simulink model "six_plus_six_AcmsteeringV09_main_2lfrf"  (R2014a)
settings: Solver=FixedStepDiscrete  StartTime=0.0  StopTime=10.0  FixedStep=0.0005  RelTol=1e-3
InitFcn:
  | Veh_Par_wxt
undefined symbols (not defined in the file or in its folder): acc_spdctl, ag_thr, B, bra_em, bra_pre_gz2, bra_pre_gz34, bra_pre_yd, brakepre_dem_data, brakeTrq_dem_data, bratrq_max, ecucoder_acal, eff_tran, ESP_switch, G, guzhang_lf, guzhang_lm, guzhang_lr, guzhang_rf, guzhang_rm, guzhang_rr, kd1, kd2, ki1, ki2, kp1, kp2, L, myFIS, premax, Radius, RC_switch, s_opt_yi, s_opt_zhuan, s_opt_zhuan_add, s_opt_zhuan_table, spd_map_mot, spd_spdctl, speed_thr_park, TCS_switch, tras_ratio, trq_map_mot, trqmax_yd, trqmax_zx, trqmaxneg, v_gain, v_table, v_thr_park, zhidong_bianmazhi, zhidong_down, zhidong_up, zhidong_youmen, zhuanxiang_bianmazhi, zhuanxiang_down, zhuanxiang_up, zhuanxiang_youmen
libraries: simulink x980, ec5744lib x59, fuzblock x2
(part 25 of 25)

== matlab function six_plus_six_AcmsteeringV09_main_2lfrf/MainControl/mode_control/forward/forward/Drive/容错控制/MATLAB Function ==
  data: trq_dem_l input; trq_dem_lf output; trq_dem_lm output; trq_dem_r input; trqlim_lf input; trqlim_lm input; trqlim_lr input; trqlim_rf input; trqlim_rm input; trqlim_rr input; guzhang_lf input; guzhang_lm input; guzhang_lr input; guzhang_rf input; guzhang_rm input; guzhang_rr input; trq_dem_lr output; trq_dem_rf output; trq_dem_rm output; trq_dem_rr output; bra_pre_l output; bra_pre_r output; bra_pre_gz2 input; bra_pre_gz34 input; mode output int8
function [trq_dem_lf,trq_dem_lm,trq_dem_lr,trq_dem_rf,trq_dem_rm,trq_dem_rr,bra_pre_l,bra_pre_r,mode] = fcn(trq_dem_l,trq_dem_r,trqlim_lf,trqlim_lm,trqlim_lr,trqlim_rf,trqlim_rm,trqlim_rr,guzhang_lf,guzhang_lm,guzhang_lr,guzhang_rf,guzhang_rm,guzhang_rr,bra_pre_gz2,bra_pre_gz34)
%#codegen
if guzhang_lf==0 && guzhang_lm==0 && guzhang_lr==0 && guzhang_rf==0 && guzhang_rm==0 && guzhang_rr==0    %0电机故障,平均分配
    trq_dem_lf=single(trq_dem_l/3);
    trq_dem_lm=single(trq_dem_l/3);
    trq_dem_lr=single(trq_dem_l/3);
    trq_dem_rf=single(trq_dem_r/3);
    trq_dem_rm=single(trq_dem_r/3);
    trq_dem_rr=single(trq_dem_r/3);
    bra_pre_l=single(0);
    bra_pre_r=single(0);
    mode=int8(1);
    
    
    
    
elseif guzhang_lf==1 && guzhang_lm==0 && guzhang_lr==0 && guzhang_rf==0 && guzhang_rm==0 && guzhang_rr==0    %1电机故障，同侧电机进行力矩转移，超过限值后，对侧亦降扭。  左前
    trq_dem_lf=single(0);
    trq_dem_lm=single(min(trq_dem_l/2,trqlim_lm));
    trq_dem_lr=single(min(trq_dem_l/2,trqlim_lr));
    trq_dem_rf=single((trq_dem_r-(trq_dem_l-trq_dem_lm-trq_dem_lr))/3);
    trq_dem_rm=single((trq_dem_r-(trq_dem_l-trq_dem_lm-trq_dem_lr))/3);
    trq_dem_rr=single((trq_dem_r-(trq_dem_l-trq_dem_lm-trq_dem_lr))/3);
    bra_pre_l=single(0);
    bra_pre_r=single(0);
    mode=int8(2);
elseif guzhang_lf==0 && guzhang_lm==1 && guzhang_lr==0 && guzhang_rf==0 && guzhang_rm==0 && guzhang_rr==0    %1电机故障，同侧电机进行力矩转移，超过限值后，对侧亦降扭。 左中
    trq_dem_lf=single(min(trq_dem_l/2,trqlim_lf));
    trq_dem_lm=single(0);
    trq_dem_lr=single(min(trq_dem_l/2,trqlim_lr));
    trq_dem_rf=single((trq_dem_r-(trq_dem_l-trq_dem_lf-trq_dem_lr))/3);
    trq_dem_rm=single((trq_dem_r-(trq_dem_l-trq_dem_lf-trq_dem_lr))/3);
    trq_dem_rr=single((trq_dem_r-(trq_dem_l-trq_dem_lf-trq_dem_lr))/3);
    bra_pre_l=single(0);
    bra_pre_r=single(0);
    mode=int8(3);
elseif guzhang_lf==0 && guzhang_lm==0 && guzhang_lr==1 && guzhang_rf==0 && guzhang_rm==0 && guzhang_rr==0    %1电机故障，同侧电机进行力矩转移，超过限值后，对侧亦降扭。 左后
    trq_dem_lf=single(min(trq_dem_l/2,trqlim_lf));
    trq_dem_lm=single(min(trq_dem_l/2,trqlim_lm));
    trq_dem_lr=single(0);
    trq_dem_rf=single((trq_dem_r-(trq_dem_l-trq_dem_lf-trq_dem_lm))/3);
    trq_dem_rm=single((trq_dem_r-(trq_dem_l-trq_dem_lf-trq_dem_lm))/3);
    trq_dem_rr=single((trq_dem_r-(trq_dem_l-trq_dem_lf-trq_dem_lm))/3);
    bra_pre_l=single(0);
    bra_pre_r=single(0);
    mode=int8(4);
elseif guzhang_lf==0 && guzhang_lm==0 && guzhang_lr==0 && guzhang_rf==1 && guzhang_rm==0 && guzhang_rr==0    %1电机故障，同侧电机进行力矩转移，超过限值后，对侧亦降扭。  右前
    trq_dem_rf=single(0);
    trq_dem_rm=single(min(trq_dem_r/2,trqlim_rm));
    trq_dem_rr=single(min(trq_dem_r/2,trqlim_rr));
    trq_dem_lf=single((trq_dem_l-(trq_dem_r-trq_dem_rm-trq_dem_rr))/3);
    trq_dem_lm=single((trq_dem_l-(trq_dem_r-trq_dem_rm-trq_dem_rr))/3);
    trq_dem_lr=single((trq_dem_l-(trq_dem_r-trq_dem_rm-trq_dem_rr))/3);
    bra_pre_l=single(0);
    bra_pre_r=single(0);
    mode=int8(5);
elseif guzhang_lf==0 && guzhang_lm==0 && guzhang_lr==0 && guzhang_rf==0 && guzhang_rm==1 && guzhang_rr==0    %1电机故障，同侧电机进行力矩转移，超过限值后，对侧亦降扭。 右中
    trq_dem_rf=single(min(trq_dem_r/2,trqlim_rf));
    trq_dem_rm=single(0);
    trq_dem_rr=single(min(trq_dem_r/2,trqlim_rr));
    trq_dem_lf=single((trq_dem_l-(trq_dem_r-trq_dem_rf-trq_dem_rr))/3);
    trq_dem_lm=single((trq_dem_l-(trq_dem_r-trq_dem_rf-trq_dem_rr))/3);
    trq_dem_lr=single((trq_dem_l-(trq_dem_r-trq_dem_rf-trq_dem_rr))/3);
    bra_pre_l=single(0);
    bra_pre_r=single(0);
    mode=int8(6);
elseif guzhang_lf==0 && guzhang_lm==0 && guzhang_lr==0 && guzhang_rf==0 && guzhang_rm==0 && guzhang_rr==1    %1电机故障，同侧电机进行力矩转移，超过限值后，对侧亦降扭。 右后
    trq_dem_rf=single(min(trq_dem_r/2,trqlim_rf));
    trq_dem_rm=single(min(trq_dem_r/2,trqlim_rm));
    trq_dem_rr=single(0);
    trq_dem_lf=single((trq_dem_l-(trq_dem_r-trq_dem_rf-trq_dem_rm))/3);
    trq_dem_lm=single((trq_dem_l-(trq_dem_r-trq_dem_rf-trq_dem_rm))/3);
    trq_dem_lr=single((trq_dem_l-(trq_dem_r-trq_dem_rf-trq_dem_rm))/3);
    bra_pre_l=single(0);
    bra_pre_r=single(0);
    mode=int8(7);
    
    
    
    
    
    
elseif guzhang_lf==1 && guzhang_lm==1 && guzhang_lr==0 && guzhang_rf==0 && guzhang_rm==0 && guzhang_rr==0    %2电机故障，同侧电机进行力矩转移，超过限值后，对侧亦降扭。  左前 左中   左侧
    trq_dem_lf=single(0);
    trq_dem_lm=single(0);
    trq_dem_lr=single(min(trq_dem_l,trqlim_lr));
    trq_dem_rf=single((trq_dem_r-(trq_dem_l-trq_dem_lr))/3);
    trq_dem_rm=single((trq_dem_r-(trq_dem_l-trq_dem_lr))/3);
    trq_dem_rr=single((trq_dem_r-(trq_dem_l-trq_dem_lr))/3);
    bra_pre_l=single(0);
    bra_pre_r=single(0);
    mode=int8(8);
elseif guzhang_lf==1 && guzhang_lm==0 && guzhang_lr==1 && guzhang_rf==0 && guzhang_rm==0 && guzhang_rr==0    %2电机故障，同侧电机进行力矩转移，超过限值后，对侧亦降扭。  左前 左后
    trq_dem_lf=single(0);
    trq_dem_lm=single(min(trq_dem_l,trqlim_lm));
    trq_dem_lr=single(0);
    trq_dem_rf=single((trq_dem_r-(trq_dem_l-trq_dem_lm))/3);
    trq_dem_rm=single((trq_dem_r-(trq_dem_l-trq_dem_lm))/3);
    trq_dem_rr=single((trq_dem_r-(trq_dem_l-trq_dem_lm))/3);
    bra_pre_l=single(0);
    bra_pre_r=single(0);
    mode=int8(9);
elseif guzhang_lf==0 && guzhang_lm==1 && guzhang_lr==1 && guzhang_rf==0 && guzhang_rm==0 && guzhang_rr==0    %2电机故障，同侧电机进行力矩转移，超过限值后，对侧亦降扭。  左中 左后
    trq_dem_lf=single(min(trq_dem_l,trqlim_lf));
    trq_dem_lm=single(0);
    trq_dem_lr=single(0);
    trq_dem_rf=single((trq_dem_r-(trq_dem_l-trq_dem_lf))/3);
    trq_dem_rm=single((trq_dem_r-(trq_dem_l-trq_dem_lf))/3);
    trq_dem_rr=single((trq_dem_r-(trq_dem_l-trq_dem_lf))/3);
    bra_pre_l=single(0);
    bra_pre_r=single(0);
    mode=int8(10);
    
elseif guzhang_lf==0 && guzhang_lm==0 && guzhang_lr==0 && guzhang_rf==1 && guzhang_rm==1 && guzhang_rr==0    %2电机故障，同侧电机进行力矩转移，超过限值后，对侧亦降扭。  右前 右中   右侧
    trq_dem_rf=single(0);
    trq_dem_rm=single(0);
    trq_dem_rr=single(min(trq_dem_r,trqlim_rr));
    trq_dem_lf=single((trq_dem_l-(trq_dem_r-trq_dem_rr))/3);
    trq_dem_lm=single((trq_dem_l-(trq_dem_r-trq_dem_rr))/3);
    trq_dem_lr=single((trq_dem_l-(trq_dem_r-trq_dem_rr))/3);
    bra_pre_l=single(0);
    bra_pre_r=single(0);
    mode=int8(11);
elseif guzhang_lf==0 && guzhang_lm==0 && guzhang_lr==0 && guzhang_rf==1 && guzhang_rm==0 && guzhang_rr==1    %2电机故障，同侧电机进行力矩转移，超过限值后，对侧亦降扭。  右前 右后
    trq_dem_rf=single(0);
    trq_dem_rm=single(min(trq_dem_r,trqlim_rm));
    trq_dem_rr=single(0);
    trq_dem_lf=single((trq_dem_l-(trq_dem_r-trq_dem_rm))/3);
    trq_dem_lm=single((trq_dem_l-(trq_dem_r-trq_dem_rm))/3);
    trq_dem_lr=single((trq_dem_l-(trq_dem_r-trq_dem_rm))/3);
    bra_pre_l=single(0);
    bra_pre_r=single(0);
    mode=int8(12);
elseif guzhang_lf==0 && guzhang_lm==0 && guzhang_lr==0 && guzhang_rf==0 && guzhang_rm==1 && guzhang_rr==1    %2电机故障，同侧电机进行力矩转移，超过限值后，对侧亦降扭。  右中 右后
    trq_dem_rf=single(min(trq_dem_r,trqlim_rf));
    trq_dem_rm=single(0);
    trq_dem_rr=single(0);
    trq_dem_lf=single((trq_dem_l-(trq_dem_r-trq_dem_rf))/3);
    trq_dem_lm=single((trq_dem_l-(trq_dem_r-trq_dem_rf))/3);
    trq_dem_lr=single((trq_dem_l-(trq_dem_r-trq_dem_rf))/3);
    bra_pre_l=single(0);
    bra_pre_r=single(0);
    mode=int8(13);
    
elseif guzhang_lf==1 && guzhang_lm==0 && guzhang_lr==0 && guzhang_rf==1 && guzhang_rm==0 && guzhang_rr==0    %2电机故障，同侧电机进行力矩转移，超过限值后，对侧亦降扭。  左前-右前 对侧
    trq_dem_lf=single(0);
    trq_dem_rf=single(0);
    trq_dem_lm=single(min(trq_dem_l/2,trqlim_lm));
    trq_dem_lr=single(min(trq_dem_l/2,trqlim_lr));
    trq_dem_rm=single(min(trq_dem_r/2,trqlim_rm));
    trq_dem_rr=single(min(trq_dem_r/2,trqlim_rr));
    if (trq_dem_l-trq_dem_lm-trq_dem_lr)>=(trq_dem_r-trq_dem_rm-trq_dem_rr)
        trq_dem_rm=single(min(trqlim_rm,(trq_dem_r-(trq_dem_l-trq_dem_lm-trq_dem_lr))/2));
        trq_dem_rr=single(min(trqlim_rr,(trq_dem_r-(trq_dem_l-trq_dem_lm-trq_dem_lr))/2));
    else
        trq_dem_lm=single(min(trqlim_lm,(trq_dem_l-(trq_dem_r-trq_dem_rm-trq_dem_rr))/2));
        trq_dem_lr=single(min(trqlim_lr,(trq_dem_l-(trq_dem_r-trq_dem_rm-trq_dem_rr))/2));
    end
    bra_pre_l=single(0);
    bra_pre_r=single(0);
    mode=int8(14);
elseif guzhang_lf==1 && guzhang_lm==0 && guzhang_lr==0 && guzhang_rf==0 && guzhang_rm==1 && guzhang_rr==0    %2电机故障，同侧电机进行力矩转移，超过限值后，对侧亦降扭。  左前-右中
    trq_dem_lf=single(0);
    trq_dem_rm=single(0);
    trq_dem_lm=single(min(trq_dem_l/2,trqlim_lm));
    trq_dem_lr=single(min(trq_dem_l/2,trqlim_lr));
    trq_dem_rf=single(min(trq_dem_r/2,trqlim_rf));
    trq_dem_rr=single(min(trq_dem_r/2,trqlim_rr));
    if (trq_dem_l-trq_dem_lm-trq_dem_lr)>=(trq_dem_r-trq_dem_rf-trq_dem_rr)
        trq_dem_rf=single(min(trqlim_rf,(trq_dem_r-(trq_dem_l-trq_dem_lm-trq_dem_lr))/2));
        trq_dem_rr=single(min(trqlim_rr,(trq_dem_r-(trq_dem_l-trq_dem_lm-trq_dem_lr))/2));
    else
        trq_dem_lm=single(min(trqlim_lm,(trq_dem_l-(trq_dem_r-trq_dem_rf-trq_dem_rr))/2));
        trq_dem_lr=single(min(trqlim_lr,(trq_dem_l-(trq_dem_r-trq_dem_rf-trq_dem_rr))/2));
    end
    bra_pre_l=single(0);
    bra_pre_r=single(0);
    mode=int8(15);
elseif guzhang_lf==1 && guzhang_lm==0 && guzhang_lr==0 && guzhang_rf==0 && guzhang_rm==0 && guzhang_rr==1    %2电机故障，同侧电机进行力矩转移，超过限值后，对侧亦降扭。  左前-右后
    trq_dem_lf=single(0);
    trq_dem_rr=single(0);
    trq_dem_lm=single(min(trq_dem_l/2,trqlim_lm));
    trq_dem_lr=single(min(trq_dem_l/2,trqlim_lr));
    trq_dem_rf=single(min(trq_dem_r/2,trqlim_rf));
    trq_dem_rm=single(min(trq_dem_r/2,trqlim_rm));
    if (trq_dem_l-trq_dem_lm-trq_dem_lr)>=(trq_dem_r-trq_dem_rf-trq_dem_rm)
        trq_dem_rf=single(min(trqlim_rf,(trq_dem_r-(trq_dem_l-trq_dem_lm-trq_dem_lr))/2));
        trq_dem_rm=single(min(trqlim_rm,(trq_dem_r-(trq_dem_l-trq_dem_lm-trq_dem_lr))/2));
    else
        trq_dem_lm=single(min(trqlim_lm,(trq_dem_l-(trq_dem_r-trq_dem_rf-trq_dem_rm))/2));
        trq_dem_lr=single(min(trqlim_lr,(trq_dem_l-(trq_dem_r-trq_dem_rf-trq_dem_rm))/2));
    end
    bra_pre_l=single(0);
    bra_pre_r=single(0);
    mode=int8(16);
    
elseif guzhang_lf==0 && guzhang_lm==1 && guzhang_lr==0 && guzhang_rf==1 && guzhang_rm==0 && guzhang_rr==0    %2电机故障，同侧电机进行力矩转移，超过限值后，对侧亦降扭。  左中-右前
    trq_dem_lm=single(0);
    trq_dem_rf=single(0);
    trq_dem_lf=single(min(trq_dem_l/2,trqlim_lf));
    trq_dem_lr=single(min(trq_dem_l/2,trqlim_lr));
    trq_dem_rm=single(min(trq_dem_r/2,trqlim_rm));
    trq_dem_rr=single(min(trq_dem_r/2,trqlim_rr));
    if (trq_dem_l-trq_dem_lf-trq_dem_lr)>=(trq_dem_r-trq_dem_rm-trq_dem_rr)
        trq_dem_rm=single(min(trqlim_rm,(trq_dem_r-(trq_dem_l-trq_dem_lf-trq_dem_lr))/2));
        trq_dem_rr=single(min(trqlim_rr,(trq_dem_r-(trq_dem_l-trq_dem_lf-trq_dem_lr))/2));
    else
        trq_dem_lf=single(min(trqlim_lf,(trq_dem_l-(trq_dem_r-trq_dem_rm-trq_dem_rr))/2));
        trq_dem_lr=single(min(trqlim_lr,(trq_dem_l-(trq_dem_r-trq_dem_rm-trq_dem_rr))/2));
    end
    bra_pre_l=single(0);
    bra_pre_r=single(0);
    mode=int8(17);
elseif guzhang_lf==0 && guzhang_lm==1 && guzhang_lr==0 && guzhang_rf==0 && guzhang_rm==1 && guzhang_rr==0    %2电机故障，同侧电机进行力矩转移，超过限值后，对侧亦降扭。  左中-右中
    trq_dem_lm=single(0);
    trq_dem_rm=single(0);
    trq_dem_lf=single(min(trq_dem_l/2,trqlim_lf));
    trq_dem_lr=single(min(trq_dem_l/2,trqlim_lr));
    trq_dem_rf=single(min(trq_dem_r/2,trqlim_rf));
    trq_dem_rr=single(min(trq_dem_r/2,trqlim_rr));
    if (trq_dem_l-trq_dem_lf-trq_dem_lr)>=(trq_dem_r-trq_dem_rf-trq_dem_rr)
        trq_dem_rf=single(min(trqlim_rf,(trq_dem_r-(trq_dem_l-trq_dem_lf-trq_dem_lr))/2));
        trq_dem_rr=single(min(trqlim_rr,(trq_dem_r-(trq_dem_l-trq_dem_lf-trq_dem_lr))/2));
    else
        trq_dem_lf=single(min(trqlim_lf,(trq_dem_l-(trq_dem_r-trq_dem_rf-trq_dem_rr))/2));
        trq_dem_lr=single(min(trqlim_lr,(trq_dem_l-(trq_dem_r-trq_dem_rf-trq_dem_rr))/2));
    end
    bra_pre_l=single(0);
    bra_pre_r=single(0);
    mode=int8(18);
elseif guzhang_lf==0 && guzhang_lm==1 && guzhang_lr==0 && guzhang_rf==0 && guzhang_rm==0 && guzhang_rr==1    %2电机故障，同侧电机进行力矩转移，超过限值后，对侧亦降扭。  左中-右后
    trq_dem_lm=single(0);
    trq_dem_rr=single(0);
    trq_dem_lf=single(min(trq_dem_l/2,trqlim_lf));
    trq_dem_lr=single(min(trq_dem_l/2,trqlim_lr));
    trq_dem_rf=single(min(trq_dem_r/2,trqlim_rf));
    trq_dem_rm=single(min(trq_dem_r/2,trqlim_rm));
    if (trq_dem_l-trq_dem_lf-trq_dem_lr)>=(trq_dem_r-trq_dem_rf-trq_dem_rm)
        trq_dem_rf=single(min(trqlim_rf,(trq_dem_r-(trq_dem_l-trq_dem_lf-trq_dem_lr))/2));
        trq_dem_rm=single(min(trqlim_rm,(trq_dem_r-(trq_dem_l-trq_dem_lf-trq_dem_lr))/2));
    else
        trq_dem_lf=single(min(trqlim_lf,(trq_dem_l-(trq_dem_r-trq_dem_rf-trq_dem_rm))/2));
        trq_dem_lr=single(min(trqlim_lr,(trq_dem_l-(trq_dem_r-trq_dem_rf-trq_dem_rm))/2));
    end
    bra_pre_l=single(0);
    bra_pre_r=single(0);
    mode=int8(19);
    
elseif guzhang_lf==0 && guzhang_lm==0 && guzhang_lr==1 && guzhang_rf==1 && guzhang_rm==0 && guzhang_rr==0    %2电机故障，同侧电机进行力矩转移，超过限值后，对侧亦降扭。  左后-右前
    trq_dem_lr=single(0);
    trq_dem_rf=single(0);
    trq_dem_lf=single(min(trq_dem_l/2,trqlim_lf));
    trq_dem_lm=single(min(trq_dem_l/2,trqlim_lm));
    trq_dem_rm=single(min(trq_dem_r/2,trqlim_rm));
    trq_dem_rr=single(min(trq_dem_r/2,trqlim_rr));
    if (trq_dem_l-trq_dem_lf-trq_dem_lm)>=(trq_dem_r-trq_dem_rm-trq_dem_rr)
        trq_dem_rm=single(min(trqlim_rm,(trq_dem_r-(trq_dem_l-trq_dem_lf-trq_dem_lm))/2));
        trq_dem_rr=single(min(trqlim_rr,(trq_dem_r-(trq_dem_l-trq_dem_lf-trq_dem_lm))/2));
    else
        trq_dem_lf=single(min(trqlim_lf,(trq_dem_l-(trq_dem_r-trq_dem_rm-trq_dem_rr))/2));
        trq_dem_lm=single(min(trqlim_lm,(trq_dem_l-(trq_dem_r-trq_dem_rm-trq_dem_rr))/2));
    end
    bra_pre_l=single(0);
    bra_pre_r=single(0);
    mode=int8(20);
elseif guzhang_lf==0 && guzhang_lm==0 && guzhang_lr==1 && guzhang_rf==0 && guzhang_rm==1 && guzhang_rr==0    %2电机故障，同侧电机进行力矩转移，超过限值后，对侧亦降扭。  左后-右中
    trq_dem_lr=single(0);
    trq_dem_rm=single(0);
    trq_dem_lf=single(min(trq_dem_l/2,trqlim_lf));
    trq_dem_lm=single(min(trq_dem_l/2,trqlim_lm));
    trq_dem_rf=single(min(trq_dem_r/2,trqlim_rf));
    trq_dem_rr=single(min(trq_dem_r/2,trqlim_rr));
    if (trq_dem_l-trq_dem_lf-trq_dem_lm)>=(trq_dem_r-trq_dem_rf-trq_dem_rr)
        trq_dem_rf=single(min(trqlim_rf,(trq_dem_r-(trq_dem_l-trq_dem_lf-trq_dem_lm))/2));
        trq_dem_rr=single(min(trqlim_rr,(trq_dem_r-(trq_dem_l-trq_dem_lf-trq_dem_lm))/2));
    else
        trq_dem_lf=single(min(trqlim_lf,(trq_dem_l-(trq_dem_r-trq_dem_rf-trq_dem_rr))/2));
        trq_dem_lm=single(min(trqlim_lm,(trq_dem_l-(trq_dem_r-trq_dem_rf-trq_dem_rr))/2));
    end
    bra_pre_l=single(0);
    bra_pre_r=single(0);
    mode=int8(21);
elseif guzhang_lf==0 && guzhang_lm==0 && guzhang_lr==1 && guzhang_rf==0 && guzhang_rm==0 && guzhang_rr==1    %2电机故障，同侧电机进行力矩转移，超过限值后，对侧亦降扭。  左后-右后
    trq_dem_lr=single(0);
    trq_dem_rr=single(0);
    trq_dem_lf=single(min(trq_dem_l/2,trqlim_lf));
    trq_dem_lm=single(min(trq_dem_l/2,trqlim_lm));
    trq_dem_rf=single(min(trq_dem_r/2,trqlim_rf));
    trq_dem_rm=single(min(trq_dem_r/2,trqlim_rm));
    if (trq_dem_l-trq_dem_lf-trq_dem_lm)>=(trq_dem_r-trq_dem_rf-trq_dem_rm)
        trq_dem_rf=single(min(trqlim_rf,(trq_dem_r-(trq_dem_l-trq_dem_lf-trq_dem_lm))/2));
        trq_dem_rm=single(min(trqlim_rm,(trq_dem_r-(trq_dem_l-trq_dem_lf-trq_dem_lm))/2));
    else
        trq_dem_lf=single(min(trqlim_lf,(trq_dem_l-(trq_dem_r-trq_dem_rf-trq_dem_rm))/2));
        trq_dem_lm=single(min(trqlim_lm,(trq_dem_l-(trq_dem_r-trq_dem_rf-trq_dem_rm))/2));
    end
    bra_pre_l=single(0);
    bra_pre_r=single(0);
    mode=int8(22);
    
    
    
    
    
    
    
    
    
elseif guzhang_lf==1 && guzhang_lm==1 && guzhang_lr==1 && guzhang_rf==0 && guzhang_rm==0 && guzhang_rr==0    %3电机故障，同侧电机进行力矩转移，超过限值后，对侧亦降扭。  左前 左中 左后   左侧
    trq_dem_lf=single(0);
    trq_dem_lm=single(0);
    trq_dem_lr=single(0);
    trq_dem_rf=single(0);
    trq_dem_rm=single(0);
    trq_dem_rr=single(0);
    bra_pre_l=single(bra_pre_gz2);
    bra_pre_r=single(bra_pre_gz2);
    mode=int8(23);
elseif guzhang_lf==0 && guzhang_lm==0 && guzhang_lr==0 && guzhang_rf==1 && guzhang_rm==1 && guzhang_rr==1    %3电机故障，同侧电机进行力矩转移，超过限值后，对侧亦降扭。  右前 右中 右后   右侧
    trq_dem_lf=single(0);
    trq_dem_lm=single(0);
    trq_dem_lr=single(0);
    trq_dem_rf=single(0);
    trq_dem_rm=single(0);
    trq_dem_rr=single(0);
    bra_pre_l=single(bra_pre_gz2);
    bra_pre_r=single(bra_pre_gz2);
    mode=int8(24);
    
elseif guzhang_lf==1 && guzhang_lm==1 && guzhang_lr==0 && guzhang_rf==1 && guzhang_rm==0 && guzhang_rr==0    %3电机故障，同侧电机进行力矩转移，超过限值后，对侧亦降扭。  左前-左中-右前 对侧
    trq_dem_lf=single(0);
    trq_dem_lm=single(0);
    trq_dem_rf=single(0);
    trq_dem_lr=single(min(trq_dem_l,trqlim_lr));
    trq_dem_rm=single(min(trq_dem_r/2,trqlim_rm));
    trq_dem_rr=single(min(trq_dem_r/2,trqlim_rr));
    if (trq_dem_l-trq_dem_lr)>=(trq_dem_r-trq_dem_rm-trq_dem_rr)
        trq_dem_rm=single(min(trqlim_rm,(trq_dem_r-(trq_dem_l-trq_dem_lr))/2));
        trq_dem_rr=single(min(trqlim_rr,(trq_dem_r-(trq_dem_l-trq_dem_lr))/2));
    else
        trq_dem_lr=single(min(trqlim_lr,(trq_dem_l-(trq_dem_r-trq_dem_rm-trq_dem_rr))));
    end
    bra_pre_l=single(0);
    bra_pre_r=single(0);
    mode=int8(25);
elseif guzhang_lf==1 && guzhang_lm==1 && guzhang_lr==0 && guzhang_rf==0 && guzhang_rm==1 && guzhang_rr==0    %3电机故障，同侧电机进行力矩转移，超过限值后，对侧亦降扭。  左前-左中-右中 对侧
    trq_dem_lf=single(0);
    trq_dem_lm=single(0);
    trq_dem_rm=single(0);
    trq_dem_lr=single(min(trq_dem_l,trqlim_lr));
    trq_dem_rf=single(min(trq_dem_r/2,trqlim_rf));
    trq_dem_rr=single(min(trq_dem_r/2,trqlim_rr));
    if (trq_dem_l-trq_dem_lr)>=(trq_dem_r-trq_dem_rf-trq_dem_rr)
        trq_dem_rf=single(min(trqlim_rf,(trq_dem_r-(trq_dem_l-trq_dem_lr))/2));
        trq_dem_rr=single(min(trqlim_rr,(trq_dem_r-(trq_dem_l-trq_dem_lr))/2));
    else
        trq_dem_lr=single(min(trqlim_lr,(trq_dem_l-(trq_dem_r-trq_dem_rf-trq_dem_rr))));
    end
    bra_pre_l=single(0);
    bra_pre_r=single(0);
    mode=int8(26);
elseif guzhang_lf==1 && guzhang_lm==1 && guzhang_lr==0 && guzhang_rf==0 && guzhang_rm==0 && guzhang_rr==1    %3电机故障，同侧电机进行力矩转移，超过限值后，对侧亦降扭。  左前-左中-右后 对侧
    trq_dem_lf=single(0);
    trq_dem_lm=single(0);
    trq_dem_rr=single(0);
    trq_dem_lr=single(min(trq_dem_l,trqlim_lr));
    trq_dem_rf=single(min(trq_dem_r/2,trqlim_rf));
    trq_dem_rm=single(min(trq_dem_r/2,trqlim_rm));
    if (trq_dem_l-trq_dem_lr)>=(trq_dem_r-trq_dem_rf-trq_dem_rm)
        trq_dem_rf=single(min(trqlim_rf,(trq_dem_r-(trq_dem_l-trq_dem_lr))/2));
        trq_dem_rm=single(min(trqlim_rm,(trq_dem_r-(trq_dem_l-trq_dem_lr))/2));
    else
        trq_dem_lr=single(min(trqlim_lr,(trq_dem_l-(trq_dem_r-trq_dem_rf-trq_dem_rm))));
    end
    bra_pre_l=single(0);
    bra_pre_r=single(0);
    mode=int8(27);
    
elseif guzhang_lf==1 && guzhang_lm==0 && guzhang_lr==1 && guzhang_rf==1 && guzhang_rm==0 && guzhang_rr==0    %3电机故障，同侧电机进行力矩转移，超过限值后，对侧亦降扭。  左前-左后-右前 对侧
    trq_dem_lf=single(0);
    trq_dem_lr=single(0);
    trq_dem_rf=single(0);
    trq_dem_lm=single(min(trq_dem_l,trqlim_lm));
    trq_dem_rm=single(min(trq_dem_r/2,trqlim_rm));
    trq_dem_rr=single(min(trq_dem_r/2,trqlim_rr));
    if (trq_dem_l-trq_dem_lm)>=(trq_dem_r-trq_dem_rm-trq_dem_rr)
        trq_dem_rm=single(min(trqlim_rm,(trq_dem_r-(trq_dem_l-trq_dem_lm))/2));
        trq_dem_rr=single(min(trqlim_rr,(trq_dem_r-(trq_dem_l-trq_dem_lm))/2));
    else
        trq_dem_lm=single(min(trqlim_lm,(trq_dem_l-(trq_dem_r-trq_dem_rm-trq_dem_rr))));
    end
    bra_pre_l=single(0);
    bra_pre_r=single(0);
    mode=int8(28);
elseif guzhang_lf==1 && guzhang_lm==0 && guzhang_lr==1 && guzhang_rf==0 && guzhang_rm==1 && guzhang_rr==0    %3电机故障，同侧电机进行力矩转移，超过限值后，对侧亦降扭。  左前-左后-右中 对侧
    trq_dem_lf=single(0);
    trq_dem_lr=single(0);
    trq_dem_rm=single(0);
    trq_dem_lm=single(min(trq_dem_l,trqlim_lm));
    trq_dem_rf=single(min(trq_dem_r/2,trqlim_rf));
    trq_dem_rr=single(min(trq_dem_r/2,trqlim_rr));
    if (trq_dem_l-trq_dem_lm)>=(trq_dem_r-trq_dem_rf-trq_dem_rr)
        trq_dem_rf=single(min(trqlim_rf,(trq_dem_r-(trq_dem_l-trq_dem_lm))/2));
        trq_dem_rr=single(min(trqlim_rr,(trq_dem_r-(trq_dem_l-trq_dem_lm))/2));
    else
        trq_dem_lm=single(min(trqlim_lm,(trq_dem_l-(trq_dem_r-trq_dem_rf-trq_dem_rr))));
    end
    bra_pre_l=single(0);
    bra_pre_r=single(0);
    mode=int8(29);
elseif guzhang_lf==1 && guzhang_lm==0 && guzhang_lr==1 && guzhang_rf==0 && guzhang_rm==0 && guzhang_rr==1    %3电机故障，同侧电机进行力矩转移，超过限值后，对侧亦降扭。  左前-左后-右后 对侧
    trq_dem_lf=single(0);
    trq_dem_lr=single(0);
    trq_dem_rr=single(0);
    trq_dem_lm=single(min(trq_dem_l,trqlim_lm));
    trq_dem_rf=single(min(trq_dem_r/2,trqlim_rf));
    trq_dem_rm=single(min(trq_dem_r/2,trqlim_rm));
    if (trq_dem_l-trq_dem_lm)>=(trq_dem_r-trq_dem_rf-trq_dem_rm)
        trq_dem_rf=single(min(trqlim_rf,(trq_dem_r-(trq_dem_l-trq_dem_lm))/2));
        trq_dem_rm=single(min(trqlim_rm,(trq_dem_r-(trq_dem_l-trq_dem_lm))/2));
    else
        trq_dem_lm=single(min(trqlim_lm,(trq_dem_l-(trq_dem_r-trq_dem_rf-trq_dem_rm))));
    end
    bra_pre_l=single(0);
    bra_pre_r=single(0);
    mode=int8(30);
    
elseif guzhang_lf==0 && guzhang_lm==1 && guzhang_lr==1 && guzhang_rf==1 && guzhang_rm==0 && guzhang_rr==0    %3电机故障，同侧电机进行力矩转移，超过限值后，对侧亦降扭。  左中-左后-右前 对侧
    trq_dem_lm=single(0);
    trq_dem_lr=single(0);
    trq_dem_rf=single(0);
    trq_dem_lf=single(min(trq_dem_l,trqlim_lf));
    trq_dem_rm=single(min(trq_dem_r/2,trqlim_rm));
    trq_dem_rr=single(min(trq_dem_r/2,trqlim_rr));
    if (trq_dem_l-trq_dem_lf)>=(trq_dem_r-trq_dem_rm-trq_dem_rr)
        trq_dem_rm=single(min(trqlim_rm,(trq_dem_r-(trq_dem_l-trq_dem_lf))/2));
        trq_dem_rr=single(min(trqlim_rr,(trq_dem_r-(trq_dem_l-trq_dem_lf))/2));
    else
        trq_dem_lf=single(min(trqlim_lf,(trq_dem_l-(trq_dem_r-trq_dem_rm-trq_dem_rr))));
    end
    bra_pre_l=single(0);
    bra_pre_r=single(0);
    mode=int8(31);
elseif guzhang_lf==0 && guzhang_lm==1 && guzhang_lr==1 && guzhang_rf==0 && guzhang_rm==1 && guzhang_rr==0    %3电机故障，同侧电机进行力矩转移，超过限值后，对侧亦降扭。  左中-左后-右中 对侧
    trq_dem_lm=single(0);
    trq_dem_lr=single(0);
    trq_dem_rm=single(0);
    trq_dem_lf=single(min(trq_dem_l,trqlim_lf));
    trq_dem_rf=single(min(trq_dem_r/2,trqlim_rf));
    trq_dem_rr=single(min(trq_dem_r/2,trqlim_rr));
    if (trq_dem_l-trq_dem_lf)>=(trq_dem_r-trq_dem_rf-trq_dem_rr)
        trq_dem_rf=single(min(trqlim_rf,(trq_dem_r-(trq_dem_l-trq_dem_lf))/2));
        trq_dem_rr=single(min(trqlim_rr,(trq_dem_r-(trq_dem_l-trq_dem_lf))/2));
    else
        trq_dem_lf=single(min(trqlim_lf,(trq_dem_l-(trq_dem_r-trq_dem_rf-trq_dem_rr))));
    end
    bra_pre_l=single(0);
    bra_pre_r=single(0);
    mode=int8(32);
elseif guzhang_lf==0 && guzhang_lm==1 && guzhang_lr==1 && guzhang_rf==0 && guzhang_rm==0 && guzhang_rr==1    %3电机故障，同侧电机进行力矩转移，超过限值后，对侧亦降扭。  左中-左后-右后 对侧
    trq_dem_lm=single(0);
    trq_dem_lr=single(0);
    trq_dem_rr=single(0);
    trq_dem_lf=single(min(trq_dem_l,trqlim_lf));
    trq_dem_rf=single(min(trq_dem_r/2,trqlim_rf));
    trq_dem_rm=single(min(trq_dem_r/2,trqlim_rm));
    if (trq_dem_l-trq_dem_lf)>=(trq_dem_r-trq_dem_rf-trq_dem_rm)
        trq_dem_rf=single(min(trqlim_rf,(trq_dem_r-(trq_dem_l-trq_dem_lf))/2));
        trq_dem_rm=single(min(trqlim_rm,(trq_dem_r-(trq_dem_l-trq_dem_lf))/2));
    else
        trq_dem_lf=single(min(trqlim_lf,(trq_dem_l-(trq_dem_r-trq_dem_rf-trq_dem_rm))));
    end
    bra_pre_l=single(0);
    bra_pre_r=single(0);
    mode=int8(33);
    
elseif guzhang_lf==1 && guzhang_lm==0 && guzhang_lr==0 && guzhang_rf==1 && guzhang_rm==1 && guzhang_rr==0    %3电机故障，同侧电机进行力矩转移，超过限值后，对侧亦降扭。  右前-右中-左前 对侧
    trq_dem_rf=single(0);
    trq_dem_rm=single(0);
    trq_dem_lf=single(0);
    trq_dem_rr=single(min(trq_dem_r,trqlim_rr));
    trq_dem_lm=single(min(trq_dem_l/2,trqlim_lm));
    trq_dem_lr=single(min(trq_dem_l/2,trqlim_lr));
    if (trq_dem_r-trq_dem_rr)>=(trq_dem_l-trq_dem_lm-trq_dem_lr)
        trq_dem_lm=single(min(trqlim_lm,(trq_dem_l-(trq_dem_r-trq_dem_rr))/2));
        trq_dem_lr=single(min(trqlim_lr,(trq_dem_l-(trq_dem_r-trq_dem_rr))/2));
    else
        trq_dem_rr=single(min(trqlim_rr,(trq_dem_r-(trq_dem_l-trq_dem_lm-trq_dem_lr))));
    end
    bra_pre_l=single(0);
    bra_pre_r=single(0);
    mode=int8(34);
elseif guzhang_lf==0 && guzhang_lm==1 && guzhang_lr==0 && guzhang_rf==1 && guzhang_rm==1 && guzhang_rr==0    %3电机故障，同侧电机进行力矩转移，超过限值后，对侧亦降扭。  右前-右中-左中 对侧
    trq_dem_rf=single(0);
    trq_dem_rm=single(0);
    trq_dem_lm=single(0);
    trq_dem_rr=single(min(trq_dem_r,trqlim_rr));
    trq_dem_lf=single(min(trq_dem_l/2,trqlim_lf));
    trq_dem_lr=single(min(trq_dem_l/2,trqlim_lr));
    if (trq_dem_r-trq_dem_rr)>=(trq_dem_l-trq_dem_lf-trq_dem_lr)
        trq_dem_lf=single(min(trqlim_lf,(trq_dem_l-(trq_dem_r-trq_dem_rr))/2));
        trq_dem_lr=single(min(trqlim_lr,(trq_dem_l-(trq_dem_r-trq_dem_rr))/2));
    else
        trq_dem_rr=single(min(trqlim_rr,(trq_dem_r-(trq_dem_l-trq_dem_lf-trq_dem_lr))));
    end
    bra_pre_l=single(0);
    bra_pre_r=single(0);
    mode=int8(35);
elseif guzhang_lf==0 && guzhang_lm==0 && guzhang_lr==1 && guzhang_rf==1 && guzhang_rm==1 && guzhang_rr==0    %3电机故障，同侧电机进行力矩转移，超过限值后，对侧亦降扭。  右前-右中-左后 对侧
    trq_dem_rf=single(0);
    trq_dem_rm=single(0);
    trq_dem_lr=single(0);
    trq_dem_rr=single(min(trq_dem_r,trqlim_rr));
    trq_dem_lf=single(min(trq_dem_l/2,trqlim_lf));
    trq_dem_lm=single(min(trq_dem_l/2,trqlim_lm));
    if (trq_dem_r-trq_dem_rr)>=(trq_dem_l-trq_dem_lf-trq_dem_lm)
        trq_dem_lf=single(min(trqlim_lf,(trq_dem_l-(trq_dem_r-trq_dem_rr))/2));
        trq_dem_lm=single(min(trqlim_lm,(trq_dem_l-(trq_dem_r-trq_dem_rr))/2));
    else
        trq_dem_rr=single(min(trqlim_rr,(trq_dem_r-(trq_dem_l-trq_dem_lf-trq_dem_lm))));
    end
    bra_pre_l=single(0);
    bra_pre_r=single(0);
    mode=int8(36);
    
elseif guzhang_lf==1 && guzhang_lm==0 && guzhang_lr==0 && guzhang_rf==1 && guzhang_rm==0 && guzhang_rr==1    %3电机故障，同侧电机进行力矩转移，超过限值后，对侧亦降扭。  右前-右后-左前 对侧
    trq_dem_rf=single(0);
    trq_dem_rr=single(0);
    trq_dem_lf=single(0);
    trq_dem_rm=single(min(trq_dem_r,trqlim_rm));
    trq_dem_lm=single(min(trq_dem_l/2,trqlim_lm));
    trq_dem_lr=single(min(trq_dem_l/2,trqlim_lr));
    if (trq_dem_r-trq_dem_rm)>=(trq_dem_l-trq_dem_lm-trq_dem_lr)
        trq_dem_lm=single(min(trqlim_lm,(trq_dem_l-(trq_dem_r-trq_dem_rm))/2));
        trq_dem_lr=single(min(trqlim_lr,(trq_dem_l-(trq_dem_r-trq_dem_rm))/2));
    else
        trq_dem_rm=single(min(trqlim_rm,(trq_dem_r-(trq_dem_l-trq_dem_lm-trq_dem_lr))));
    end
    bra_pre_l=single(0);
    bra_pre_r=single(0);
    mode=int8(37);
elseif guzhang_lf==0 && guzhang_lm==1 && guzhang_lr==0 && guzhang_rf==1 && guzhang_rm==0 && guzhang_rr==1    %3电机故障，同侧电机进行力矩转移，超过限值后，对侧亦降扭。  右前-右后-左中 对侧
    trq_dem_rf=single(0);
    trq_dem_rr=single(0);
    trq_dem_lm=single(0);
    trq_dem_rm=single(min(trq_dem_r,trqlim_rm));
    trq_dem_lf=single(min(trq_dem_l/2,trqlim_lf));
    trq_dem_lr=single(min(trq_dem_l/2,trqlim_lr));
    if (trq_dem_r-trq_dem_rm)>=(trq_dem_l-trq_dem_lf-trq_dem_lr)
        trq_dem_lf=single(min(trqlim_lf,(trq_dem_l-(trq_dem_r-trq_dem_rm))/2));
        trq_dem_lr=single(min(trqlim_lr,(trq_dem_l-(trq_dem_r-trq_dem_rm))/2));
    else
        trq_dem_rm=single(min(trqlim_rm,(trq_dem_r-(trq_dem_l-trq_dem_lf-trq_dem_lr))));
    end
    bra_pre_l=single(0);
    bra_pre_r=single(0);
    mode=int8(38);
elseif guzhang_lf==0 && guzhang_lm==0 && guzhang_lr==1 && guzhang_rf==1 && guzhang_rm==0 && guzhang_rr==1    %3电机故障，同侧电机进行力矩转移，超过限值后，对侧亦降扭。  右前-右后-左后 对侧
    trq_dem_rf=single(0);
    trq_dem_rr=single(0);
    trq_dem_lr=single(0);
    trq_dem_rm=single(min(trq_dem_r,trqlim_rm));
    trq_dem_lf=single(min(trq_dem_l/2,trqlim_lf));
    trq_dem_lm=single(min(trq_dem_l/2,trqlim_lm));
    if (trq_dem_r-trq_dem_rm)>=(trq_dem_l-trq_dem_lf-trq_dem_lm)
        trq_dem_lf=single(min(trqlim_lf,(trq_dem_l-(trq_dem_r-trq_dem_rm))/2));
        trq_dem_lm=single(min(trqlim_lm,(trq_dem_l-(trq_dem_r-trq_dem_rm))/2));
    else
        trq_dem_rm=single(min(trqlim_rm,(trq_dem_r-(trq_dem_l-trq_dem_lf-trq_dem_lm))));
    end
    bra_pre_l=single(0);
    bra_pre_r=single(0);
    mode=int8(39);
    
elseif guzhang_lf==1 && guzhang_lm==0 && guzhang_lr==0 && guzhang_rf==0 && guzhang_rm==1 && guzhang_rr==1    %3电机故障，同侧电机进行力矩转移，超过限值后，对侧亦降扭。  右中-右后-左前 对侧
    trq_dem_rm=single(0);
    trq_dem_rr=single(0);
    trq_dem_lf=single(0);
    trq_dem_rf=single(min(trq_dem_r,trqlim_rf));
    trq_dem_lm=single(min(trq_dem_l/2,trqlim_lm));
    trq_dem_lr=single(min(trq_dem_l/2,trqlim_lr));
    if (trq_dem_r-trq_dem_rf)>=(trq_dem_l-trq_dem_lm-trq_dem_lr)
        trq_dem_lm=single(min(trqlim_lm,(trq_dem_l-(trq_dem_r-trq_dem_rf))/2));
        trq_dem_lr=single(min(trqlim_lr,(trq_dem_l-(trq_dem_r-trq_dem_rf))/2));
    else
        trq_dem_rf=single(min(trqlim_rf,(trq_dem_r-(trq_dem_l-trq_dem_lm-trq_dem_lr))));
    end
    bra_pre_l=single(0);
    bra_pre_r=single(0);
    mode=int8(40);
elseif guzhang_lf==0 && guzhang_lm==1 && guzhang_lr==0 && guzhang_rf==0 && guzhang_rm==1 && guzhang_rr==1    %3电机故障，同侧电机进行力矩转移，超过限值后，对侧亦降扭。  右中-右后-左中 对侧
    trq_dem_rm=single(0);
    trq_dem_rr=single(0);
    trq_dem_lm=single(0);
    trq_dem_rf=single(min(trq_dem_r,trqlim_rf));
    trq_dem_lf=single(min(trq_dem_l/2,trqlim_lf));
    trq_dem_lr=single(min(trq_dem_l/2,trqlim_lr));
    if (trq_dem_r-trq_dem_rf)>=(trq_dem_l-trq_dem_lf-trq_dem_lr)
        trq_dem_lf=single(min(trqlim_lf,(trq_dem_l-(trq_dem_r-trq_dem_rf))/2));
        trq_dem_lr=single(min(trqlim_lr,(trq_dem_l-(trq_dem_r-trq_dem_rf))/2));
    else
        trq_dem_rf=single(min(trqlim_rf,(trq_dem_r-(trq_dem_l-trq_dem_lf-trq_dem_lr))));
    end
    bra_pre_l=single(0);
    bra_pre_r=single(0);
    mode=int8(41);
elseif guzhang_lf==0 && guzhang_lm==0 && guzhang_lr==1 && guzhang_rf==0 && guzhang_rm==1 && guzhang_rr==1    %3电机故障，同侧电机进行力矩转移，超过限值后，对侧亦降扭。  右中-右后-左后 对侧
    trq_dem_rm=single(0);
    trq_dem_rr=single(0);
    trq_dem_lr=single(0);
    trq_dem_rf=single(min(trq_dem_r,trqlim_rf));
    trq_dem_lf=single(min(trq_dem_l/2,trqlim_lf));
    trq_dem_lm=single(min(trq_dem_l/2,trqlim_lm));
    if (trq_dem_r-trq_dem_rf)>=(trq_dem_l-trq_dem_lf-trq_dem_lm)
        trq_dem_lf=single(min(trqlim_lf,(trq_dem_l-(trq_dem_r-trq_dem_rf))/2));
        trq_dem_lm=single(min(trqlim_lm,(trq_dem_l-(trq_dem_r-trq_dem_rf))/2));
    else
        trq_dem_rf=single(min(trqlim_rf,(trq_dem_r-(trq_dem_l-trq_dem_lf-trq_dem_lm))));
    end
    bra_pre_l=single(0);
    bra_pre_r=single(0);
    mode=int8(42);
    
    
    
    
    
    
    
    
    
    
    
    
    
    
elseif (guzhang_lf==1 && guzhang_lm==1 && guzhang_lr==1 && guzhang_rf==1 && guzhang_rm==0 && guzhang_rr==0) || (guzhang_lf==1 && guzhang_lm==1 && guzhang_lr==1 && guzhang_rf==0 && guzhang_rm==1 && guzhang_rr==0) || (guzhang_lf==1 && guzhang_lm==1 && guzhang_lr==1 && guzhang_rf==0 && guzhang_rm==0 && guzhang_rr==1)    %4电机故障，同侧电机进行力矩转移，超过限值后，对侧亦降扭。  左前 左中 左后 右前/右中/右后   左侧
    trq_dem_lf=single(0);
    trq_dem_lm=single(0);
    trq_dem_lr=single(0);
    trq_dem_rf=single(0);
    trq_dem_rm=single(0);
    trq_dem_rr=single(0);
    bra_pre_l=single(bra_pre_gz2);
    bra_pre_r=single(bra_pre_gz2);
    mode=int8(43);
elseif (guzhang_lf==1 && guzhang_lm==0 && guzhang_lr==0 && guzhang_rf==1 && guzhang_rm==1 && guzhang_rr==1) || (guzhang_lf==0 && guzhang_lm==1 && guzhang_lr==0 && guzhang_rf==1 && guzhang_rm==1 && guzhang_rr==1) || (guzhang_lf==0 && guzhang_lm==0 && guzhang_lr==1 && guzhang_rf==1 && guzhang_rm==1 && guzhang_rr==1)   %4电机故障，同侧电机进行力矩转移，超过限值后，对侧亦降扭。  右前 右中 右后 左前/左中/左后   右侧
    trq_dem_lf=single(0);
    trq_dem_lm=single(0);
    trq_dem_lr=single(0);
    trq_dem_rf=single(0);
    trq_dem_rm=single(0);
    trq_dem_rr=single(0);
    bra_pre_l=single(bra_pre_gz2);
    bra_pre_r=single(bra_pre_gz2);
    mode=int8(44);
    
elseif guzhang_lf==1 && guzhang_lm==1 && guzhang_lr==0 && guzhang_rf==1 && guzhang_rm==1 && guzhang_rr==0    %4电机故障，同侧电机进行力矩转移，超过限值后，对侧亦降扭。  左前-左中-右前-右中 对侧
    trq_dem_lf=single(0);
    trq_dem_lm=single(0);
    trq_dem_rf=single(0);
    trq_dem_rm=single(0);
    trq_dem_lr=single(min(trq_dem_l,trqlim_lr));
    trq_dem_rr=single(min(trq_dem_r,trqlim_rr));
    if (trq_dem_l-trq_dem_lr)>=(trq_dem_r-trq_dem_rr)
        trq_dem_rr=single(min(trqlim_rr,(trq_dem_r-(trq_dem_l-trq_dem_lr))));
    else
        trq_dem_lr=single(min(trqlim_lr,(trq_dem_l-(trq_dem_r-trq_dem_rr))));
    end
    bra_pre_l=single(0);
    bra_pre_r=single(0);
    mode=int8(45);
elseif guzhang_lf==1 && guzhang_lm==1 && guzhang_lr==0 && guzhang_rf==1 && guzhang_rm==0 && guzhang_rr==1    %4电机故障，同侧电机进行力矩转移，超过限值后，对侧亦降扭。  左前-左中-右前-右后 对侧
    trq_dem_lf=single(0);
    trq_dem_lm=single(0);
    trq_dem_rf=single(0);
    trq_dem_rr=single(0);
    trq_dem_lr=single(min(trq_dem_l,trqlim_lr));
    trq_dem_rm=single(min(trq_dem_r,trqlim_rm));
    if (trq_dem_l-trq_dem_lr)>=(trq_dem_r-trq_dem_rm)
        trq_dem_rm=single(min(trqlim_rm,(trq_dem_r-(trq_dem_l-trq_dem_lr))));
    else
        trq_dem_lr=single(min(trqlim_lr,(trq_dem_l-(trq_dem_r-trq_dem_rm))));
    end
    bra_pre_l=single(0);
    bra_pre_r=single(0);
    mode=int8(46);
elseif guzhang_lf==1 && guzhang_lm==1 && guzhang_lr==0 && guzhang_rf==0 && guzhang_rm==1 && guzhang_rr==1    %4电机故障，同侧电机进行力矩转移，超过限值后，对侧亦降扭。  左前-左中-右中-右后 对侧
    trq_dem_lf=single(0);
    trq_dem_lm=single(0);
    trq_dem_rm=single(0);
    trq_dem_rr=single(0);
    trq_dem_lr=single(min(trq_dem_l,trqlim_lr));
    trq_dem_rf=single(min(trq_dem_r,trqlim_rf));
    if (trq_dem_l-trq_dem_lr)>=(trq_dem_r-trq_dem_rf)
        trq_dem_rf=single(min(trqlim_rf,(trq_dem_r-(trq_dem_l-trq_dem_lr))));
    else
        trq_dem_lr=single(min(trqlim_lr,(trq_dem_l-(trq_dem_r-trq_dem_rf))));
    end
    bra_pre_l=single(0);
    bra_pre_r=single(0);
    mode=int8(47);
    
elseif guzhang_lf==1 && guzhang_lm==0 && guzhang_lr==1 && guzhang_rf==1 && guzhang_rm==1 && guzhang_rr==0    %4电机故障，同侧电机进行力矩转移，超过限值后，对侧亦降扭。  左前-左后-右前-右中 对侧
    trq_dem_lf=single(0);
    trq_dem_lr=single(0);
    trq_dem_rf=single(0);
    trq_dem_rm=single(0);
    trq_dem_lm=single(min(trq_dem_l,trqlim_lm));
    trq_dem_rr=single(min(trq_dem_r,trqlim_rr));
    if (trq_dem_l-trq_dem_lm)>=(trq_dem_r-trq_dem_rr)
        trq_dem_rr=single(min(trqlim_rr,(trq_dem_r-(trq_dem_l-trq_dem_lm))));
    else
        trq_dem_lm=single(min(trqlim_lm,(trq_dem_l-(trq_dem_r-trq_dem_rr))));
    end
    bra_pre_l=single(0);
    bra_pre_r=single(0);
    mode=int8(48);
elseif guzhang_lf==1 && guzhang_lm==0 && guzhang_lr==1 && guzhang_rf==1 && guzhang_rm==0 && guzhang_rr==1    %4电机故障，同侧电机进行力矩转移，超过限值后，对侧亦降扭。  左前-左后-右前-右后 对侧
    trq_dem_lf=single(0);
    trq_dem_lr=single(0);
    trq_dem_rf=single(0);
    trq_dem_rr=single(0);
    trq_dem_lm=single(min(trq_dem_l,trqlim_lm));
    trq_dem_rm=single(min(trq_dem_r,trqlim_rm));
    if (trq_dem_l-trq_dem_lm)>=(trq_dem_r-trq_dem_rm)
        trq_dem_rm=single(min(trqlim_rm,(trq_dem_r-(trq_dem_l-trq_dem_lm))));
    else
        trq_dem_lm=single(min(trqlim_lm,(trq_dem_l-(trq_dem_r-trq_dem_rm))));
    end
    bra_pre_l=single(0);
    bra_pre_r=single(0);
    mode=int8(49);
elseif guzhang_lf==1 && guzhang_lm==0 && guzhang_lr==1 && guzhang_rf==0 && guzhang_rm==1 && guzhang_rr==1    %4电机故障，同侧电机进行力矩转移，超过限值后，对侧亦降扭。  左前-左后-右中-右后 对侧
    trq_dem_lf=single(0);
    trq_dem_lr=single(0);
    trq_dem_rm=single(0);
    trq_dem_rr=single(0);
    trq_dem_lm=single(min(trq_dem_l,trqlim_lm));
    trq_dem_rf=single(min(trq_dem_r,trqlim_rf));
    if (trq_dem_l-trq_dem_lm)>=(trq_dem_r-trq_dem_rf)
        trq_dem_rf=single(min(trqlim_rf,(trq_dem_r-(trq_dem_l-trq_dem_lm))));
    else
        trq_dem_lm=single(min(trqlim_lm,(trq_dem_l-(trq_dem_r-trq_dem_rf))));
    end
    bra_pre_l=single(0);
    bra_pre_r=single(0);
    mode=int8(50);
    
elseif guzhang_lf==0 && guzhang_lm==1 && guzhang_lr==1 && guzhang_rf==1 && guzhang_rm==1 && guzhang_rr==0    %4电机故障，同侧电机进行力矩转移，超过限值后，对侧亦降扭。  左中-左后-右前-右中 对侧
    trq_dem_lm=single(0);
    trq_dem_lr=single(0);
    trq_dem_rf=single(0);
    trq_dem_rm=single(0);
    trq_dem_lf=single(min(trq_dem_l,trqlim_lf));
    trq_dem_rr=single(min(trq_dem_r,trqlim_rr));
    if (trq_dem_l-trq_dem_lf)>=(trq_dem_r-trq_dem_rr)
        trq_dem_rr=single(min(trqlim_rr,(trq_dem_r-(trq_dem_l-trq_dem_lf))));
    else
        trq_dem_lf=single(min(trqlim_lf,(trq_dem_l-(trq_dem_r-trq_dem_rr))));
    end
    bra_pre_l=single(0);
    bra_pre_r=single(0);
    mode=int8(51);
elseif guzhang_lf==0 && guzhang_lm==1 && guzhang_lr==1 && guzhang_rf==1 && guzhang_rm==0 && guzhang_rr==1    %4电机故障，同侧电机进行力矩转移，超过限值后，对侧亦降扭。  左中-左后-右前-右后 对侧
    trq_dem_lm=single(0);
    trq_dem_lr=single(0);
    trq_dem_rf=single(0);
    trq_dem_rr=single(0);
    trq_dem_lf=single(min(trq_dem_l,trqlim_lf));
    trq_dem_rm=single(min(trq_dem_r,trqlim_rm));
    if (trq_dem_l-trq_dem_lf)>=(trq_dem_r-trq_dem_rm)
        trq_dem_rm=single(min(trqlim_rm,(trq_dem_r-(trq_dem_l-trq_dem_lf))));
    else
        trq_dem_lf=single(min(trqlim_lf,(trq_dem_l-(trq_dem_r-trq_dem_rm))));
    end
    bra_pre_l=single(0);
    bra_pre_r=single(0);
    mode=int8(52);
elseif guzhang_lf==0 && guzhang_lm==1 && guzhang_lr==1 && guzhang_rf==0 && guzhang_rm==1 && guzhang_rr==1    %4电机故障，同侧电机进行力矩转移，超过限值后，对侧亦降扭。  左中-左后-右中-右后 对侧
    trq_dem_lm=single(0);
    trq_dem_lr=single(0);
    trq_dem_rm=single(0);
    trq_dem_rr=single(0);
    trq_dem_lf=single(min(trq_dem_l,trqlim_lf));
    trq_dem_rf=single(min(trq_dem_r,trqlim_rf));
    if (trq_dem_l-trq_dem_lf)>=(trq_dem_r-trq_dem_rf)
        trq_dem_rf=single(min(trqlim_rf,(trq_dem_r-(trq_dem_l-trq_dem_lf))));
    else
        trq_dem_lf=single(min(trqlim_lf,(trq_dem_l-(trq_dem_r-trq_dem_rf))));
    end
    bra_pre_l=single(0);
    bra_pre_r=single(0);
    mode=int8(53);
    
    
    
    
    
    
    
    
    
    
    
    
elseif (guzhang_lf==0 && guzhang_lm==1 && guzhang_lr==1 && guzhang_rf==1 && guzhang_rm==1 && guzhang_rr==1) || (guzhang_lf==1 && guzhang_lm==0 && guzhang_lr==1 && guzhang_rf==1 && guzhang_rm==1 && guzhang_rr==1) || (guzhang_lf==1 && guzhang_lm==1 && guzhang_lr==0 && guzhang_rf==1 && guzhang_rm==1 && guzhang_rr==1) || (guzhang_lf==1 && guzhang_lm==1 && guzhang_lr==1 && guzhang_rf==0 && guzhang_rm==1 && guzhang_rr==1) || (guzhang_lf==1 && guzhang_lm==1 && guzhang_lr==1 && guzhang_rf==1 && guzhang_rm==0 && guzhang_rr==1) || (guzhang_lf==1 && guzhang_lm==1 && guzhang_lr==1 && guzhang_rf==1 && guzhang_rm==1 && guzhang_rr==0)  %5电机故障，同侧电机进行力矩转移，超过限值后，对侧亦降扭。  左前 左中 左后 右前/右中/右后   左侧
    trq_dem_lf=single(0);
    trq_dem_lm=single(0);
    trq_dem_lr=single(0);
    trq_dem_rf=single(0);
    trq_dem_rm=single(0);
    trq_dem_rr=single(0);
    bra_pre_l=single(bra_pre_gz2);
    bra_pre_r=single(bra_pre_gz2);
    mode=int8(54);
    
    
    
    
    
    
    
else    %6电机故障，同侧电机进行力矩转移，超过限值后，对侧亦降扭。  左前 左中 左后 右前/右中/右后   左侧
    trq_dem_lf=single(0);
    trq_dem_lm=single(0);
    trq_dem_lr=single(0);
    trq_dem_rf=single(0);
    trq_dem_rm=single(0);
    trq_dem_rr=single(0);
    bra_pre_l=single(bra_pre_gz2);
    bra_pre_r=single(bra_pre_gz2);
    mode=int8(55);
end
    
    
    
    
    
    
    
    % trq_dem_lf=max(0,trq_dem_lf);%电机转矩不小于0，就是不能出现负值
    % trq_dem_lr=max(0,trq_dem_lr);
    % trq_dem_rf=max(0,trq_dem_rf);
    % trq_dem_rr=max(0,trq_dem_rr);
    trq_dem_lf=single(max(-trqlim_lf,trq_dem_lf));%电机转矩可以出现负值，不超过负的外特性
    trq_dem_lm=single(max(-trqlim_lm,trq_dem_lm));
    trq_dem_lr=single(max(-trqlim_lr,trq_dem_lr));
    trq_dem_rf=single(max(-trqlim_rf,trq_dem_rf));
    trq_dem_rm=single(max(-trqlim_rm,trq_dem_rm));
    trq_dem_rr=single(max(-trqlim_rr,trq_dem_rr));
    bra_pre_l=single(bra_pre_l);
    bra_pre_r=single(bra_pre_r);
end
